simulink model "quy_hoach_quy_dao"  (R2022b)
settings: Solver=FixedStepAuto  StartTime=0.0  StopTime=10  FixedStep=0.01  RelTol=1e-3
settings Model: Creator=Admin  LastModifiedBy=Admin

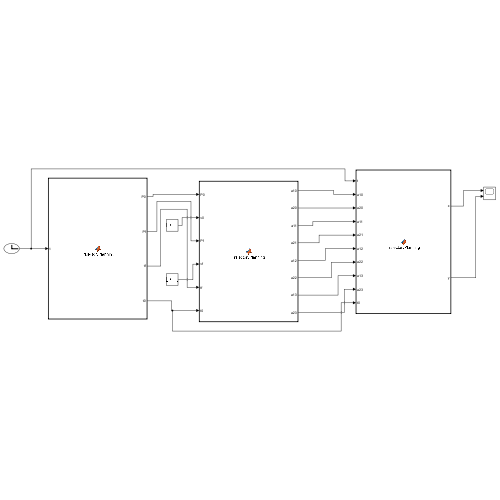
[thumbnail: Simulink's stored preview of the top-level diagram]
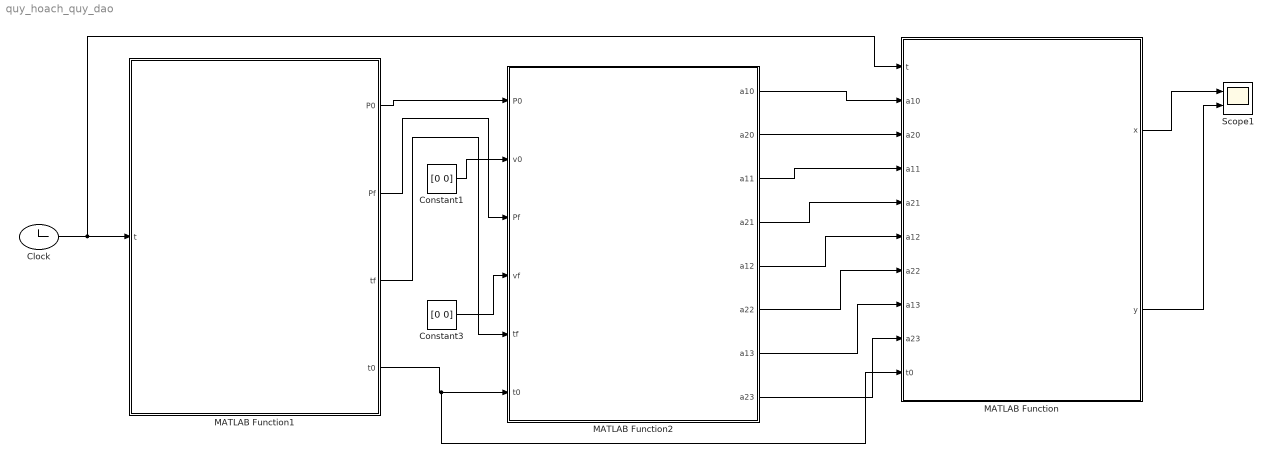
== system quy_hoach_quy_dao ==
  Clock : Clock
      settings: Decimation=20
  Constant1 : Constant  Value=[0 0]
  Constant3 : Constant  Value=[0 0]
  MATLAB Function : MATLAB Function  TreatAsAtomicUnit=on
  MATLAB Function1 : MATLAB Function  TreatAsAtomicUnit=on
  MATLAB Function2 : MATLAB Function  TreatAsAtomicUnit=on
  Scope1 : Scope  NumInputPorts=2
  wires:
  MATLAB Function/2(y) -> Scope1/2
  MATLAB Function/1(x) -> Scope1/1
  Constant3/1 -> MATLAB Function2/4(vf)
  Constant1/1 -> MATLAB Function2/2(v0)
  MATLAB Function1/1(P0) -> MATLAB Function2/1(P0)
  MATLAB Function1/2(Pf) -> MATLAB Function2/3(Pf)
  Clock/1 -> MATLAB Function/1(t), MATLAB Function1/1(t)
  MATLAB Function2/1(a10) -> MATLAB Function/2(a10)
  MATLAB Function2/2(a20) -> MATLAB Function/3(a20)
  MATLAB Function2/3(a11) -> MATLAB Function/4(a11)
  MATLAB Function2/4(a21) -> MATLAB Function/5(a21)
  MATLAB Function2/5(a12) -> MATLAB Function/6(a12)
  MATLAB Function2/6(a22) -> MATLAB Function/7(a22)
  MATLAB Function2/7(a13) -> MATLAB Function/8(a13)
  MATLAB Function2/8(a23) -> MATLAB Function/9(a23)
  MATLAB Function1/3(tf) -> MATLAB Function2/5(tf)
  MATLAB Function1/4(t0) -> MATLAB Function/10(t0), MATLAB Function2/6(t0)

== matlab function quy_hoach_quy_dao/MATLAB Function1 ==
  data: P0 output; t input; Pf output; tf output; t0 output
function [P0,Pf,tf,t0] = TrajectoryPlanning(t)
    if t <= 2
        P0 = [10;10];
        Pf = [-20;-20];
        tf = 2;
        t0 =0;
    elseif (t>= 2 && t <= 4)
        P0 = [-20;-20];
        Pf =[10;-20];
        t0 = 2;
        tf = 4;
    else
        P0 = [10;-20];
        Pf =[10;10];
        t0 = 4;
        tf = 6;
    end
 
return

== matlab function quy_hoach_quy_dao/MATLAB Function ==
  data: x output; t input; y output; a10 input; a20 input; a11 input; a21 input; a12 input; a22 input; a13 input; a23 input; t0 input
function [x,y] = TrajectoryPlanning(t,a10, a20, a11, a21, a12, a22, a13, a23, t0)
if (t<=6)
    tt=t-t0;
    x=a10+a11*tt+a12*tt^2+a13*tt^3;
    y=a20+a21*tt+a22*tt^2+a23*tt^3;
else
    x = 10;
    y = 10;
end
return

== matlab function quy_hoach_quy_dao/MATLAB Function2 ==
  data: a10 output; a20 output; P0 input; v0 input; Pf input; vf input; tf input; a11 output; a21 output; a12 output; a22 output; a13 output; a23 output; t0 input
function [a10, a20, a11, a21, a12, a22, a13, a23] = TrajectoryPlanning(P0,v0,Pf,vf,tf, t0)
    a10=P0(1);
    a20=P0(2);
    a11=v0(1);
    a21=v0(2);
    a12=3/(tf-t0)^2*(Pf(1)-P0(1))-2/(tf-t0)*v0(1)- 1/(tf-t0)*vf(1);
    a22=3/(tf-t0)^2*(Pf(2)-P0(2))-2/(tf-t0)*v0(2)- 1/(tf-t0)*vf(2);
    a13=-2/(tf-t0)^3*(Pf(1)-P0(1))+1/(tf-t0)^2*(vf(1)+v0(1));
    a23=-2/(tf-t0)^3*(Pf(2)-P0(2))+1/(tf-t0)^2*(vf(2)+v0(2));
return
